simulink model "accBasedController_Simulation"  (R2020a)
settings: Solver=VariableStepAuto  StartTime=0  StopTime=20  FixedStep=0.001  RelTol=1e-3
values from neighbouring files (symbols this model uses):
  A = [0 0 5.53191489362 0 0 0 0 -107.82412766 0 221.276595745 0 1 ... (25 elements, 5x5)]    [CACu_ws.mat]    (also in SimulationParameters.m = [0 0 0 1 0 0;      0 0 0 0 1 0;      0 0 0 0 0 1;      -Ka/J; Simulation_ws.mat = [0 0 0 -118.993135011 5.87581816357 0 0 0 0 118.993135011 -1; abc_ws.mat = [0 0 0 1828.84460673 0 0 0 0 -1965.91569285 221.276595745 0 ; kalmanSS.m = [0 0 0 1 0 0;      0 0 0 0 1 0;      0 0 0 0 0 1;      -Ka/J)
  B = [1  0; 0  0; 0  0; 0  0; 0  19.2446808511]    [CACu_ws.mat]    (also in SimulationParameters.m = [zeros(3,control_dim); 1/Jh 0 0; 0 -1/Je 0; 0 0 N*KI/Ja]; Simulation_ws.mat = [0 0 0 22.8832951945 0 0 0 0 0 0 -1.12996503145 0 ... (18 el; abc_ws.mat = [1 0 0 0 0 0 0 0 -1.31799121269 0 0 0 ... (15 elements, 5x3); kalmanSS.m = [zeros(3,control_dim); 1/Jh 0 0; 0 -1/Je 0; 0 0 N*KI/Ja])
  C = [0 0 0 0 0 0 1 0 0 0 0 0 ... (25 elements, 5x5)]    [CACu_ws.mat]    (also in SimulationParameters.m = [zeros(sensor_dim,state_dim)]; Simulation_ws.mat = [-5.2 0 0 0 0 0 5.2 0 1 0 0 0 ... (36 elements, 6x6)]; abc_ws.mat; kalmanSS.m = [zeros(sensor_dim,state_dim)])
  CURRENT_MAX = 3.14    [CAC_ws.mat]    (also in CACu_ws.mat; SimulationParameters.m = 3.14159265359; Simulation_ws.mat = 3.14159265359; TransferFunctions.m = 3.14159265359)
  D = [1  0; 0  0; 0  0; 0  0; 0  0]    [CACu_ws.mat]    (also in SimulationParameters.m = zeros(sensor_dim, control_dim); Simulation_ws.mat = [0 0 0 0 0 0 0 0 0 0 0 0 ... (18 elements, 6x3)]; abc_ws.mat = [1 0 0 0 0 0 0 0 0 0 0 0 ... (15 elements, 5x3)]; kalmanSS.m = zeros(sensor_dim, control_dim))
  damping_d = 1.6    [CAC_ws.mat]    (also in CACu_ws.mat = 0.770835010154; abc_ws.mat = 0.770835010154; kalmanSSHumInput.m = 0.9; kalmanStateSpaceModellingHumInput.m = 0.9)
  dt = 0.001    [SimulationParameters.m]    (also in Simulation_ws.mat; TransferFunctions.m; kalmanSS.m; tests_analysis.m = 0.008)
  epos_Ki = 1.19    [CAC_ws.mat]    (also in CACu_ws.mat; TransferFunctions.m; abc_ws.mat; kalmanSSHumInput.m)
  epos_Kp = 11.9    [CAC_ws.mat]    (also in CACu_ws.mat; TransferFunctions.m; abc_ws.mat; kalmanSSHumInput.m)
  Fk = eye(state_dim) + A*dt + (A*dt)^2/prod(1:2) + (A*dt)^3/prod(1:3) + (A*dt)^4/prod(1:4)    [SimulationParameters.m]    (also in Simulation_ws.mat = [0.999940504052 2.93784973961e-06 5.41742100187e-11 -0.11899; kalmanSS.m)
  Gk = dt*(eye(state_dim) + A*dt/prod(1:2) + (A*dt)^2/prod(1:3) + (A*dt)^3/prod(1:4) +         (A*dt)^4/prod(1:5))*B    [SimulationParameters.m]    (also in Simulation_ws.mat = [1.14415341408e-05 5.60242006442e-12 0 0.0228828413715 2.240; kalmanSS.m = dt*(eye(state_dim) + A*dt/prod(1:2) + (A*dt)^2/prod(1:3) + ()
  I_zz = mass_scale*body_mass*(L_leg*r_zz)^2    (= 0.0437446334976)    [KneeJointParameters.m]    (also in SimulationParameters.m; Simulation_ws.mat; TransferFunctions.m; abc_ws.mat)
  Ja = 0.47    [CACu_ws.mat]    (also in SimulationParameters.m; Simulation_ws.mat; TransferFunctions.m; abc_ws.mat)
  Je = 0.94    [CACu_ws.mat]    (also in SimulationParameters.m = 0.88498313856; Simulation_ws.mat = 0.88498313856; TransferFunctions.m = 0.88498313856; abc_ws.mat = 0.7587304)
  Jh = 0.05    [CACu_ws.mat]    (also in SimulationParameters.m = 0.0437; Simulation_ws.mat = 0.0437; TransferFunctions.m = 0.0437; abc_ws.mat = 0.0437)
  Ka = 5.2    [CACu_ws.mat]    (also in SimulationParameters.m; Simulation_ws.mat; TransferFunctions.m = 6552; abc_ws.mat = 1387.6)
  KI = 0.0603    [CACu_ws.mat]    (also in SimulationParameters.m; Simulation_ws.mat; TransferFunctions.m; abc_ws.mat)
  Ks = 104    [CACu_ws.mat]    (also in SimulationParameters.m; Simulation_ws.mat; TransferFunctions.m; abc_ws.mat)
  Le = 0.4    [CACu_ws.mat]    (also in SimulationParameters.m = 0.432; Simulation_ws.mat = 0.432; TransferFunctions.m = 0.432; abc_ws.mat)
  N = 150    [CACu_ws.mat]    (also in SimulationParameters.m; Simulation_ws.mat; TransferFunctions.m; abc_ws.mat)
  Rk = eye(sensor_dim)    [kalmanStateSpaceModellingWithoutHum.m]
  sensor_dim = 5    [CACu_ws.mat]    (also in SimulationParameters.m = 6; Simulation_ws.mat = 6; abc_ws.mat; kalmanSS.m = 6)
  state_dim = 5    [CACu_ws.mat]    (also in SimulationParameters.m = 6; Simulation_ws.mat = 6; abc_ws.mat; kalmanSS.m = 6)
  stiffness_d = 1.04    [CAC_ws.mat]    (also in CACu_ws.mat = 14.0803237251; abc_ws.mat = 14.0803237251; kalmanSSHumInput.m = 3.874; kalmanStateSpaceModellingHumInput.m = 3.874)
  stiffness_lower = -20.9019922533    [CACu_ws.mat]    (also in abc_ws.mat; kalmanSSHumInput.m = -24.4873189611; kalmanStateSpaceModellingHumInput.m = -24.4873189611)
  Threaded_Ts = 0.001    [CAC_ws.mat]    (also in CACu_ws.mat; SimulationParameters.m; Simulation_ws.mat; abc_ws.mat)
  We = 19.6133    [CACu_ws.mat]    (also in SimulationParameters.m = 46.5037717323; Simulation_ws.mat = 46.5037717323; TransferFunctions.m = 46.5037717323; abc_ws.mat = 46.5037717323)
  zeta = 0.06    [SimulationParameters.m]    (also in Simulation_ws.mat; TransferFunctions.m; abc_ws.mat; kalmanSSHumInput.m = 0.01)
undefined symbols (not defined in the file or in its folder): A_kf, alpha, B_kf, C_kf, Continuous, D_kf, DiscIntNeverNeededParam, Discrete, gamma, k_bar, kf_ste_dim, nm_window, p_e_idx, p_m_idx, rho, sigma, Time, v_e_idx, v_h_idx, v_m_idx
libraries: simulink x23, dspstat3 x8, simulink_extras x5, ctrlSharedLib x2, dspsigops x2
(part 1 of 2)
Description:
  | Collocated Admittance Control study for the acceleration-based SEA Transparency Control
settings Model: OrderedModelArguments=off  Creator=Leonardo Felipe  LastModifiedBy=leona
settings DataIOCC: LimitDataPoints=on  MaxDataPoints=23000  SaveFormat=Array  InspectSignalLogs=on  ReturnWorkspaceOutputs=off
settings SFSimCC: CustomCodeUndefinedFunction=UseInterfaceOnly

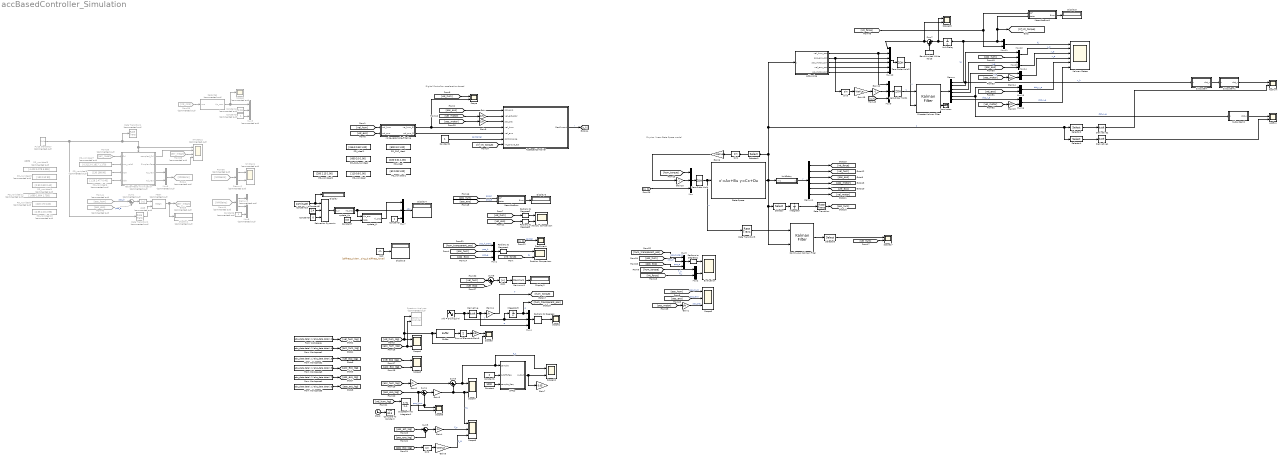
== system accBasedController_Simulation ==
  note: //RMS
  note: Digital Controller: acceleration-based
  note: Physics, linear State Space model
  Abs1 : Abs
  Abs3 : Abs  Commented=on
  AccBasedController : Subsystem  SystemSampleTime=dt
  AccExo : Scope  NumInputPorts=2
  AccHum : Scope  NumInputPorts=2
  Band-Limited White Noise : simulink/Sources/Band-Limited White Noise  Cov=2*5.476e-6  Ts=dt  seed=[23341]  VectorParams1D=off
  Buffer : Buffer  N=8  OutputFrames=off
  CAC : Constant  Value=[stiffness_d damping_d stiffness_lower]
  Clock : Clock
  Compare To Constant : simulink/Logic and Bit Operations/Compare To Constant  relop=<=  const=32.5  OutDataTypeStr=boolean
  Constant : Constant  Value=1000
  Constant1 : Constant  Value=2
  Constant10 : Constant  Value=sqrt(Ka/Je)
  Constant2 : Constant
  Constant3 : Constant  Commented=on
  Constant4 : Constant  Commented=on  Value=2.15
  Constant5 : Constant
  Constant6 : Constant  Commented=on
  Constant7 : Constant  Value=0.8
  Constant8 : Constant  Value=2.4
  Constant9 : Constant  Value=0
  Continuous Kalman Filter : ctrlSharedLib/Kalman Filter  TimeDomain=Continuous-Time  UseCurrentEstimator=on  ModelSource=LTI State-Space Variable  ModelSourceVariable=ss(A, B, C, D)  A=Fk  B=Gk  C=C  D=D  NumberOfStates=1  NumberOfInputs=1  NumberOfOutputs=1  InitialEstimateSource=Dialog  X0=zeros(state_dim,1)  P0=10  UseK=off  UseGH=off  NumberOfProcessNoiseInputs=1  G=1  TimeInvariantG=on  H=0  TimeInvariantH=on  Q=0.005*eye(state_dim)  TimeInvariantQ=on  R=0.01*eye(sensor_dim)  TimeInvariantR=on  N=0  TimeInvariantN=on  AddInputPort=on  AddEnablePort=off  OutputEstimatedY=off  OutputP=off  Ts=dt
  DIscrete Kalman Filter : ctrlSharedLib/Kalman Filter  TimeDomain=Discrete-Time  UseCurrentEstimator=on  ModelSource=Individual A, B, C, D matrices  ModelSourceVariable=ss(A_kf, B_kf, C_kf, D_kf)  A=Fk  B=Gk  C=C_kf  D=D_kf  NumberOfStates=1  NumberOfInputs=1  NumberOfOutputs=1  InitialEstimateSource=Dialog  X0=zeros(kf_ste_dim,1)  P0=10  UseK=off  UseGH=off  NumberOfProcessNoiseInputs=1  G=1  TimeInvariantG=on  H=0  TimeInvariantH=on  Q=Qk  TimeInvariantQ=on  R=Rk  TimeInvariantR=on  N=0  TimeInvariantN=on  AddInputPort=on  AddEnablePort=off  OutputEstimatedY=on  OutputP=off  Ts=dt
  Demux : Demux  Outputs=kf_ste_dim
  Demux1 : Demux  Outputs=6
  Demux2 : Demux  Commented=on  Outputs=2
  Demux3 : Demux  Commented=on  Outputs=2
  Derivative : Derivative
  Derivative1 : Derivative
  Derivative2 : Derivative
  DesCurrent : Scope
  Discrete-Time Integrator1 : DiscreteIntegrator  ExternalReset=level  InitialCondition=-0.16  SampleTime=dt  ICPrevOutput=DiscIntNeverNeededParam  ICPrevScaledInput=DiscIntNeverNeededParam
  Display{,2..6} (6 alike) : Display
  Display1 : Display  Commented=on
  Evaluation : Scope  NumInputPorts=2
  From Workspace : FromWorkspace  VariableName=[abc_data.data(:,1) abc_data.data(:,2)]  SampleTime=dt  OutputAfterFinalValue=Holding final value
  From Workspace1 : FromWorkspace  VariableName=[abc_data.data(:,1) abc_data.data(:,4)]  SampleTime=dt  OutputAfterFinalValue=Holding final value
  From Workspace2 : FromWorkspace  VariableName=[abc_data.data(:,1) abc_data.data(:,3)]  SampleTime=dt  OutputAfterFinalValue=Holding final value
  From Workspace3 : FromWorkspace  VariableName=[abc_data.data(:,1) abc_data.data(:,5)]  SampleTime=dt  OutputAfterFinalValue=Holding final value
  From Workspace4 : FromWorkspace  VariableName=[abc_data.data(:,1) abc_data.data(:,7)]  SampleTime=dt  OutputAfterFinalValue=Holding final value
  From Workspace5 : FromWorkspace  VariableName=[abc_data.data(:,1) abc_data.data(:,6)]  SampleTime=dt  OutputAfterFinalValue=Holding final value
  From35 : From  Commented=on  GotoTag=err_mean
  From36 : From  Commented=on  GotoTag=NMGains
  From38 : From  Commented=on  GotoTag=err_mean
  From39 : From  Commented=on  GotoTag=int_rms
  From40 : From  Commented=on  GotoTag=pos_exo
  From41 : From  Commented=on  GotoTag=pos_hum
  From44 : From  Commented=on  GotoTag=NMGains
  Gain{,1,8,13..14} (5 alike) : Gain  Gain=1/N
  Gain10 : Gain  Gain=-1
  Gain11 : Gain  Gain=Jh
  Gain12 : Gain  Gain=-1
  Gain15 : Gain  Gain=-We*Le
  Gain2 : Gain  Gain=Jh
  Gain3 : Gain  Gain=Ks/20
  Gain4 : Gain  Gain=Ks
  Gain5 : Gain  Gain=-We*Le
  Gain6 : Gain  Gain=-We*Le
  Gain7 : Gain  Gain=0.05
  Gain9 : Gain  Gain=1/8
  Goto4 : Goto  Commented=on  GotoTag=NMGains
  Goto5 : Goto  Commented=on  GotoTag=err_mean
  Integrator : Integrator
  Integrator3 : Integrator
  Kalman States : Scope  NumInputPorts=6
  LPF2p : Subsystem
  Maximum1 : dspstat3/Maximum  operation=maximum  fcn=Running  indexBase=One  operateOver=Each column  Dimension=1  InputProcessing=Columns as channels (frame based)  reset=None  roiEnable=off  roiType=Rectangles  roiPortion=Entire ROI  roiOutput=Individual statistics for each ROI  roiFlag=off  roundingMode=Floor  overflowMode=off  accumDataTypeStr=Inherit: Same as product output  accumLastDataTypeStr=Inherit: Same as product output
  Mean : dspstat3/Mean  Commented=on  run=on  InputProcessing=Columns as channels (frame based)  reset_popup=Falling edge  directionMode=Each column  dimension=1  roiEnable=off  roiType=Rectangles  roiPortion=Entire ROI  roiOutput=Individual statistics for each ROI  roiFlag=off  roundingMode=Floor  overflowMode=off  outputDataTypeStr=Inherit: Same as accumulator  outputMin=[]  outputMax=[]  outputLastDataTypeStr=Inherit: Same as accumulator
  MeanAbsError : Subsystem
  MeanAbsError1 : Subsystem
  Mux{,1,3..4,7,9} (6 alike) : Mux  Inputs=3
  Mux10 : Mux  Inputs=kf_snr_dim
  Mux{2,11..16} (7 alike) : Mux  Inputs=2
  Mux5 : Mux  Commented=on  Inputs=3
  Mux6 : Mux  Commented=on  Inputs=2
  Mux8 : Mux  Commented=on  Inputs=3
  NM Gains : Scope  Commented=on  NumInputPorts=2
  NM Status : Scope  Commented=on  NumInputPorts=4
  Nelder-Mead minimization : Subsystem  Commented=on  TreatAsAtomicUnit=on
  PD_CAC_ideal : Constant  Value=[600 3.0 1.00]
  PD_CAC_nonideal : Constant  Value=[600 3.0 1.00]
  PD_ideal : Constant  Value=[100 0.01 1.00]
  PD_ideal1 : Constant  Value=[246.9 0.60 1.00]
  PD_nonideal : Constant  Value=[110 0.8 1.00]
  PD_nonideal1 : Constant  Value=[60 0.08 1.00]
  PD_nonideal10 : Constant  Commented=on  Value=[2.55 2.15 2.95]  VectorParams1D=off
  PD_nonideal11 : Constant  Commented=on  Value=[1.699 1.604 1.758]
  PD_nonideal2 : Constant  Value=[200 2.15 1.00]
  PD_nonideal3 : Constant  Commented=on  Value=[130 110 90]
  PD_nonideal4 : Constant  Commented=on  Value=[0.90 0.80 0.40]  VectorParams1D=off
  PD_nonideal5 : Constant  Commented=on  Value=[130 188 90]
  PD_nonideal6 : Constant  Commented=on  Value=[1.29 2.477 0.40]  VectorParams1D=off
  PD_nonideal7 : Constant  Commented=on  Value=[0.3113 0.1817 1.170]
  PD_nonideal8 : Constant  Commented=on  Value=[4.423 5.078 6.355]
  PD_nonideal9 : Constant  Commented=on  Value=[220 170 240]
  Position Comparison : Scope  NumInputPorts=2
  Pulse Generator : DiscretePulseGenerator  Commented=on  PulseType=Time based  Period=nm_window  PulseWidth=5  PhaseDelay=0.95*nm_window
  Radians to Degrees{,1..4} (5 alike) : simulink_extras/Transformations/Radians to Degrees
  Rate Transition : RateTransition  OutPortSampleTime=dt
  Rate Transition1 : RateTransition  Commented=on
  Rate Transition2 : RateTransition  Commented=on
  Rate Transition3 : RateTransition
  Saturation Dynamic : simulink/Discontinuities/Saturation Dynamic  OutMin=[]  OutMax=[]  OutDataTypeStr=Inherit: Same as second input  OutDataType=fixdt(1, 16)  OutScaling=2^-10  DoSatur=off
  Scope{,3..5,7..8,10,17..18} (9 alike) : Scope  NumInputPorts=2
  Scope1 : Scope
  Scope2 : Scope  Commented=on
  Scope6 : Scope  NumInputPorts=3
  Scope9 : Scope  NumInputPorts=3
  Secantes : Subsystem  Commented=on  TreatAsAtomicUnit=on
  Selector : Selector  InputPortWidth=sensor_dim  IndexOptions=Index vector (dialog)  Indices=[v_h_idx]  OutputSizes=1
  Selector1 : Selector  InputPortWidth=sensor_dim  IndexOptions=Index vector (dialog)  Indices=[p_e_idx]  OutputSizes=1
  Selector2 : Selector  InputPortWidth=sensor_dim  IndexOptions=Index vector (dialog)  Indices=[v_h_idx]  OutputSizes=1
  Selector3 : Selector  InputPortWidth=state_dim  IndexOptions=Index vector (dialog)  Indices=[4]  OutputSizes=1
  Selector4 : Selector  InputPortWidth=sensor_dim  IndexOptions=Index vector (dialog)  Indices=[v_e_idx]  OutputSizes=1
  Sin1 : Trigonometry
  Sin2 : Trigonometry
  Sin3 : Trigonometry
  Spectrum Analyzer : SpectrumAnalyzer  Commented=on  NumInputPorts=2
  State-Space : StateSpace  A=A  B=B  C=C  D=D  InitialCondition=0  ContinuousStateAttributes={'x_h','x_e','x_a','dx_h','dx_e','dx_a'}
  Subsystem : Subsystem
  Subsystem1 : Subsystem
  Subsystem2 : Subsystem
  Sum of Elements : Sum  Inputs=+
  Sum1 : Sum  Commented=on  Inputs=|+-
  Sum{3..6} (4 alike) : Sum  Inputs=|+-
  Sum7 : Sum  Inputs=|++
  Terminator : Terminator
  Unit Delay : UnitDelay  SampleTime=-1  HasFrameUpgradeWarning=on
  UnitDelay : Subsystem  TreatAsAtomicUnit=on  SystemSampleTime=dt
  Velocity Comparison : Scope  NumInputPorts=2
  Zero-Order Hold : ZeroOrderHold  SampleTime=Threaded_Ts
  Zero-Order Hold1 : ZeroOrderHold  SampleTime=dt
  Zero-Order Hold2 : ZeroOrderHold  SampleTime=dt
  add_noise : Subsystem
  noise_resample_filtering : Subsystem
  update_Ki : Subsystem
  update_Kp : Subsystem
  w(t) = 3*sin(2pi*t) : Sin  Amplitude=3  Frequency=2*pi  SampleTime=0
  wires:
  Zero-Order Hold/1 -> Rate Transition3/1, State-Space/1  "u"
  State-Space/1 -> Selector4/1, Selector2/1, add_noise/1(y), Selector1/1, Selector/1, Continuous Kalman Filter/2, UnitDelay/1(In1)  "z"
  Mux/1 -> Zero-Order Hold/1
  UnitDelay/1(y) -> Demux1/1  "y"
  [vel_hum] -> Radians to Degrees2/1
  [vel_exo] -> Radians to Degrees3/1
  [pos_hum] -> Scope6/1  "pos_hum"
  [pos_exo] -> Scope6/2  "pos_exo"
  Constant2/1 -> AccBasedController/6(control_type)  "controller"
  [pos_exo] -> AccBasedController/1(pos_exo)
  [vel_motor] -> Gain/1
  Sin1/1 -> Gain6/1
  Demux1/3 -> [pos_exo]
  AccBasedController/1(DesCurrent) -> [u_k]  "I"
  Gain6/1 -> Gain10/1
  [pos_motor] -> Gain1/1
  Radians to Degrees2/1 -> Velocity Comparison/1
  Radians to Degrees3/1 -> Velocity Comparison/2
  [u_k] -> DesCurrent/1  "control"
  Gain10/1 -> Mux/2
  [vel_hum] -> Scope/1
  Demux1/2 -> [vel_hum]
  Demux1/1 -> [int_force]
  Demux1/4 -> [pos_motor]
  Demux1/5 -> [vel_exo]
  Demux1/6 -> [vel_motor]
  Mux1/1 -> Radians to Degrees4/1
  Radians to Degrees4/1 -> Position Comparison/1
  [int_force] -> Position Comparison/2  "t_i"
  [hum_torque] -> Mux/1
  Gain/1 -> AccBasedController/2(vel_actuator)
  Gain1/1 -> Scope6/3  "pos_act"
  From Workspace/1 -> [vel_hum_log]
  From Workspace1/1 -> [acc_hum_log]
  From Workspace3/1 -> [acc_exo_log]
  From Workspace2/1 -> [vel_exo_log]
  [acc_hum_log] -> Spectrum Analyzer/2, Scope4/2
  [vel_hum_log] -> Scope3/2, Buffer/1, Spectrum Analyzer/1, Scope4/1
  [acc_exo_log] -> Scope5/2
  [vel_exo_log] -> Scope5/1
  [acc_hum_log] -> Gain2/1
  Gain2/1 -> Sum3/1
  Sum4/1 -> Gain3/1
  Gain3/1 -> Sum3/2, Scope9/1, Scope7/2  "F_i"
  From Workspace4/1 -> [pos_exo_log]
  [pos_exo_log] -> Scope8/2, Sum4/1
  [vel_hum_log] -> Discrete-Time Integrator1/1
  Discrete-Time Integrator1/1 -> Sum4/2, Scope8/1  "pos_hum"
  Sum3/1 -> Scope10/1, LPF2p/1(sample), Scope7/1  "F_h"
  Clock/1 -> Compare To Constant/1
  From Workspace5/1 -> [pos_act_log]
  Sum5/1 -> Gain4/1
  [pos_act_log] -> Sum5/1
  [pos_exo_log] -> Sum5/2
  Gain4/1 -> Scope9/2  "F_s"
  Gain5/1 -> Scope9/3  "F_W"
  Sin2/1 -> Gain5/1
  [pos_exo_log] -> Sin2/1
  Constant/1 -> LPF2p/3(sample_freq)
  Constant1/1 -> LPF2p/2(cutoff_freq)
  LPF2p/1(output) -> Scope10/2, Gain7/1
  [vel_hum] -> Sum6/1
  [vel_exo] -> Sum6/2
  Abs1/1 -> Maximum1/1
  Maximum1/1 -> Display2/1
  Sum6/1 -> Abs1/1
  Gain8/1 -> AccBasedController/3(pos_act)
  [pos_motor] -> Gain8/1
  CAC/1 -> Display3/1
  Selector/1 -> Integrator/1
  Integrator/1 -> Rate Transition/1
  Rate Transition/1 -> [pos_hum]
  Selector1/1 -> Sin1/1
  [u_k] -> Mux/3
  [vel_hum] -> noise_resample_filtering/1(vel_hum)
  [vel_exo] -> noise_resample_filtering/2(vel_exo)
  noise_resample_filtering/1(ve_hum_filt) -> AccBasedController/4(vel_hum), Scope/2
  Mux3/1 -> Radians to Degrees1/1
  [pos_exo] -> Mux3/3  "pos_e"
  [pos_hum] -> Mux3/2  "pos_h"
  [hum_torque] -> Mux2/1  "T_h"
  [int_force] -> Mux2/2  "T_i"
  Mux2/1 -> Evaluation/2
  Radians to Degrees1/1 -> Evaluation/1
  [pos_exo] -> Mux1/3  "pos_e"
  [pos_hum] -> Mux1/2  "pos_h"
  [hum_transparent_pos] -> Mux1/1  "pos_h_trans"
  w(t) = 3*sin(2pi*t)/1 -> Integrator3/1, Mux4/2, Derivative/1  "v"
  Derivative/1 -> Mux4/3, Gain11/1  "a"
  Integrator3/1 -> [hum_transparent_pos], Mux4/1  "p"
  Mux4/1 -> Radians to Degrees/1
  Gain11/1 -> [hum_torque]  "T"
  Radians to Degrees/1 -> Scope1/1
  Constant3/1 -> Mux5/3
  From35/1 -> Nelder-Mead minimization/1(f(x))
  Pulse Generator/1 -> Rate Transition2/1, Rate Transition1/1, Nelder-Mead minimization/Trigger, NM Status/1
  PD_nonideal5/1 -> Nelder-Mead minimization/3(Kp0)
  PD_nonideal6/1 -> Nelder-Mead minimization/4(Kd0)
  PD_nonideal7/1 -> Nelder-Mead minimization/2(rms_vals0)
  Mux6/1 -> Goto4/1
  Nelder-Mead minimization/3(Kp_new) -> Mux6/1
  Nelder-Mead minimization/4(Kd_new) -> Mux6/2
  Nelder-Mead minimization/1(sampled_f(x)) -> NM Status/2
  From36/1 -> Demux2/1
  Demux2/1 -> NM Gains/1
  Demux2/2 -> NM Gains/2
  Nelder-Mead minimization/2(SimplexCase) -> NM Status/4
  From38/1 -> NM Status/3
  From39/1 -> Secantes/1(rms)
  Constant4/1 -> Mux5/2
  Secantes/1(Kp_new) -> Scope2/1, Mux5/1
  Constant5/1 -> Mux7/3
  From41/1 -> Sum1/1  "pos_h"
  From40/1 -> Sum1/2  "pos_e"
  Sum1/1 -> Abs3/1
  Abs3/1 -> Mean/1
  Mean/1 -> Display1/1, Goto5/1
  Rate Transition2/1 -> Mean/2
  Mux7/1 -> Display4/1  "Abc"
  Demux3/2 -> Mux8/2
  Demux3/1 -> Mux8/1
  Constant6/1 -> Mux8/3
  From44/1 -> Demux3/1
  update_Kp/1(Kp_acc) -> Mux7/2, update_Ki/1(Kp_acc)
  update_Ki/1(Ki_acc) -> Mux7/1
  Constant7/1 -> update_Ki/2(zeta)
  Constant9/1 -> Saturation Dynamic/3
  Constant8/1 -> Saturation Dynamic/2
  Saturation Dynamic/1 -> update_Kp/1(w_n)
  Constant10/1 -> Display/1, Saturation Dynamic/1
  [hum_transparent_pos] -> Mux3/1  "pos_h_trans"
  noise_resample_filtering/2(vel_exo_filt) -> AccBasedController/5(vel_exo)
  Buffer/1 -> Sum of Elements/1
  Sum of Elements/1 -> Gain9/1
  Gain9/1 -> Scope3/1
  add_noise/1(vel_hum_corr) -> Mux10/2, Mux9/1
  Gain12/1 -> Mux9/2
  Mux9/1 -> Zero-Order Hold1/1
  Zero-Order Hold1/1 -> DIscrete Kalman Filter/1  "u"
  [u_k] -> Mux9/3
  DIscrete Kalman Filter/1 -> Demux/1
  Mux10/1 -> Zero-Order Hold2/1
  add_noise/4(vel_exo_corr) -> Mux10/5
  Zero-Order Hold2/1 -> DIscrete Kalman Filter/2  "u"
  Rate Transition3/1 -> Continuous Kalman Filter/1
  Continuous Kalman Filter/1 -> Selector3/1
  Selector3/1 -> Scope17/1
  [vel_hum] -> Scope17/2
  [int_force] -> MeanAbsError1/1(ref), Mux11/2
  [pos_exo] -> Mux13/2
  Demux/3 -> Mux13/1  "x_e"
  Demux/1 -> MeanAbsError1/2(state), [kf_int_torque], Mux11/1, Unit Delay/1  "t_i"
  Demux/2 -> Mux12/1, Subsystem/1(x)  "x_h"
  [pos_hum] -> Mux12/2
  Demux/4 -> Mux14/1  "x_a"
  [pos_motor] -> Gain14/1
  Gain14/1 -> Mux14/2
  [vel_motor] -> Gain13/1
  [vel_exo] -> Mux15/2
  Demux/5 -> Mux15/1, Subsystem2/1(x)  "dot_x_e"
  Band-Limited White Noise/1 -> Sum7/2
  Sum7/1 -> Scope18/2, Mux10/1
  add_noise/2(pos_exo_corr) -> Sin3/1, Mux10/3
  add_noise/3(pos_motor_corr) -> Mux10/4
  add_noise/5(vel_motor_corr) -> Mux10/6
  Unit Delay/1 -> Scope18/1, Sum7/1
  Sin3/1 -> Gain15/1
  Gain15/1 -> Gain12/1
  Mux11/1 -> Kalman States/1  "t_i"
  Mux12/1 -> Kalman States/2  "x_h"
  Mux13/1 -> Kalman States/3  "x_e"
  Mux14/1 -> Kalman States/4  "x_a"
  Gain13/1 -> Mux16/2
  Demux/6 -> Mux16/1  "dot_x_a"
  Mux15/1 -> Kalman States/5  "dot_x_e"
  Mux16/1 -> Kalman States/6  "dot_x_a"
  [kf_int_torque] -> AccBasedController/7(int_torque_est)
  DIscrete Kalman Filter/2 -> Terminator/1
  Selector2/1 -> Derivative2/1
  Subsystem/1(dot_x) -> Subsystem1/1(x)
  Selector4/1 -> Derivative1/1
  [pos_hum] -> MeanAbsError/1(ref)  "pos_h"
  [pos_exo] -> MeanAbsError/2(state)  "pos_e"
  MeanAbsError/1(Error) -> Display6/1
  MeanAbsError1/1(Error) -> Display5/1
  Subsystem1/1(dot_x) -> AccHum/1
  Derivative2/1 -> AccHum/2
  Subsystem2/1(dot_x) -> AccExo/1
  Derivative1/1 -> AccExo/2

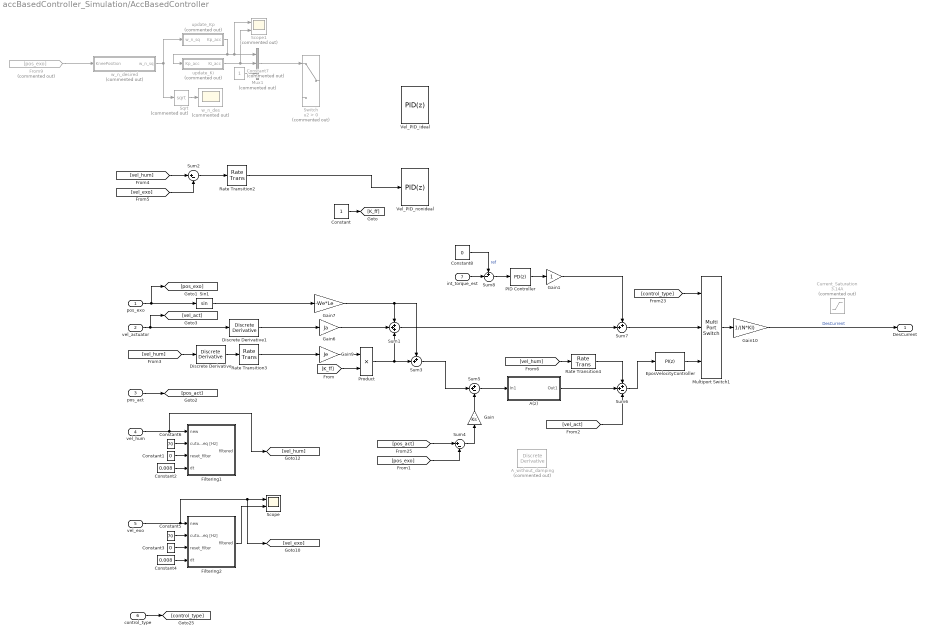
== system accBasedController_Simulation/AccBasedController ==
  pos_exo : Inport
  vel_actuator : Inport  Port=2
  pos_act : Inport  Port=3
  vel_hum : Inport  Port=4
  vel_exo : Inport  Port=5
  control_type : Inport  Port=6
  int_torque_est : Inport  Port=7
  A(z) : Subsystem
  A_without_damping : simulink/Discrete/Discrete Derivative  Commented=on  gainval=k_bar/stiffness_d  ICPrevScaledInput=0.0  OutMin=[]  OutMax=[]  OutDataType=fixdt(1, 16)  OutScaling=2^-10  DoSatur=off
  Constant : Constant
  Constant1 : Constant  Value=0
  Constant2 : Constant  Value=0.008
  Constant3 : Constant  Value=0
  Constant4 : Constant  Value=0.008
  Constant5 : Constant  Value=70
  Constant6 : Constant  Value=70
  Constant7 : Constant  Commented=on
  Constant8 : Constant  Value=0
  Current_Saturation 3.14A : Saturate  Commented=on  UpperLimit=CURRENT_MAX  LowerLimit=-CURRENT_MAX
  Discrete Derivative : simulink/Discrete/Discrete Derivative  gainval=1.0  ICPrevScaledInput=0.0  OutMin=[]  OutMax=[]  OutDataType=fixdt(1, 16)  OutScaling=2^-10  DoSatur=off
  Discrete Derivative1 : simulink/Discrete/Discrete Derivative  gainval=1.0  ICPrevScaledInput=0.0  OutMin=[]  OutMax=[]  OutDataType=fixdt(1, 16)  OutScaling=2^-10  DoSatur=off
  EposVelocityController : simulink/Continuous/PID Controller  Controller=PI  Form=Parallel  TimeDomain=Discrete-time  UseExternalTs=off  SampleTime=dt  IntegratorMethod=Forward Euler  FilterMethod=Forward Euler  ControllerParametersSource=internal  P=epos_Kp  I=epos_Ki  D=279.805559989798  UseFilter=off  N=100  TunerSelectOption=Transfer Function Based (PID Tuner App)  InitialConditionSource=internal  InitialConditionForIntegrator=0  InitialConditionForFilter=0  DifferentiatorICPrevScaledInput=0  ExternalReset=none  TrackingMode=off  Kt=1  LimitOutput=off  UpperSaturationLimit=inf  LowerSaturationLimit=-inf  LinearizeAsGain=on  AntiWindupMode=none  Kb=1  POutMin=[]  POutMax=[]  IOutMin=[]  IOutMax=[]  DOutMin=[]  DOutMax=[]  NOutMin=[]  NOutMax=[]  SumOutMin=[]  SumOutMax=[]  SaturationOutMin=[]  SaturationOutMax=[]  PParamMin=[]  PParamMax=[]  IParamMin=[]  IParamMax=[]  DParamMin=[]  DParamMax=[]  NParamMin=[]  NParamMax=[]  KbParamMin=[]  KbParamMax=[]  KtParamMin=[]  KtParamMax=[]  KbOutMin=[]  KbOutMax=[]  KtOutMin=[]  KtOutMax=[]  IntegratorOutMin=[]  IntegratorOutMax=[]  FilterOutMin=[]  FilterOutMax=[]  SumI1OutMin=[]  SumI1OutMax=[]  SumI2OutMin=[]  SumI2OutMax=[]  SumI3OutMin=[]  SumI3OutMax=[]  SumI4OutMin=[]  SumI4OutMax=[]  SumDOutMin=[]  SumDOutMax=[]  DifferentiatorOutMin=[]  DifferentiatorOutMax=[]  FilterDiffOutCoefMin=[]  FilterDiffOutCoefMax=[]  ReciprocalOutMin=[]  ReciprocalOutMax=[]  SumDenOutMin=[]  SumDenOutMax=[]  SumNumOutMin=[]  SumNumOutMax=[]  DivideOutMin=[]  DivideOutMax=[]  UdiffTsProdOutMin=[]  UdiffTsProdOutMax=[]  NTsProdOutMin=[]  NTsProdOutMax=[]  UintegralTsProdOutMin=[]  UintegralTsProdOutMax=[]  UngainTsProdOutMin=[]  UngainTsProdOutMax=[]  IntegratorContinuousStateAttributes=''  IntegratorStateMustResolveToSignalObject=off  IntegratorRTWStateStorageClass=Auto  FilterContinuousStateAttributes=''  FilterStateMustResolveToSignalObject=off  FilterRTWStateStorageClass=Auto  ParallelPVariant=InternalParameters  IdealPVariant=Disabled  IVariant=InternalParameters  DVariant=Disabled  IntegratorVariant=Discrete  SatVariant=Disabled  AWVariant=Passthrough  PCopyVariant=Disabled  TRVariant=Disabled  FdbkBlocksVariant=Forward  IdealPFdbkVariant=Disabled  SatFdbkVariant=Disabled  DerivativeFilterVariant=Disabled  NVariant=Disabled  NCopyVariant=Disabled_SignalSpec  FilterICVariant=Disabled  IntegratorICVariant=InternalICs  ExternalResetVariant=Disabled  TRSumVariant=Passthrough  SumFdbkVariant=Disabled  SumVariant=Sum_PI  TsampFilterVariant=InternalTs  TsampNgainVariant=Passthrough  TsampIntegralVariant=Passthrough
  Filtering1 : Subsystem
  Filtering2 : Subsystem
  From9 : From  Commented=on  GotoTag=pos_exo
  Gain : Gain  Gain=Ks
  Gain1 : Gain
  Gain10 : Gain  Gain=1/(N*KI)
  Gain6 : Gain  Gain=Ja
  Gain7 : Gain  Gain=-We*Le
  Gain9 : Gain  Gain=Je
  Multiport Switch1 : MultiPortSwitch  Inputs=2
  Mux1 : Mux  Commented=on  Inputs=3
  PID Controller : simulink/Continuous/PID Controller  Controller=PD  Form=Parallel  TimeDomain=Discrete-time  UseExternalTs=off  SampleTime=dt  IntegratorMethod=Forward Euler  FilterMethod=Forward Euler  ControllerParametersSource=internal  P=23  I=1  D=1.6  UseFilter=on  N=100  TunerSelectOption=Transfer Function Based (PID Tuner App)  InitialConditionSource=internal  InitialConditionForIntegrator=0  InitialConditionForFilter=0  DifferentiatorICPrevScaledInput=0  ExternalReset=none  TrackingMode=off  Kt=1  LimitOutput=off  UpperSaturationLimit=inf  LowerSaturationLimit=-inf  LinearizeAsGain=on  AntiWindupMode=none  Kb=1  POutMin=[]  POutMax=[]  IOutMin=[]  IOutMax=[]  DOutMin=[]  DOutMax=[]  NOutMin=[]  NOutMax=[]  SumOutMin=[]  SumOutMax=[]  SaturationOutMin=[]  SaturationOutMax=[]  PParamMin=[]  PParamMax=[]  IParamMin=[]  IParamMax=[]  DParamMin=[]  DParamMax=[]  NParamMin=[]  NParamMax=[]  KbParamMin=[]  KbParamMax=[]  KtParamMin=[]  KtParamMax=[]  KbOutMin=[]  KbOutMax=[]  KtOutMin=[]  KtOutMax=[]  IntegratorOutMin=[]  IntegratorOutMax=[]  FilterOutMin=[]  FilterOutMax=[]  SumI1OutMin=[]  SumI1OutMax=[]  SumI2OutMin=[]  SumI2OutMax=[]  SumI3OutMin=[]  SumI3OutMax=[]  SumI4OutMin=[]  SumI4OutMax=[]  SumDOutMin=[]  SumDOutMax=[]  DifferentiatorOutMin=[]  DifferentiatorOutMax=[]  FilterDiffOutCoefMin=[]  FilterDiffOutCoefMax=[]  ReciprocalOutMin=[]  ReciprocalOutMax=[]  SumDenOutMin=[]  SumDenOutMax=[]  SumNumOutMin=[]  SumNumOutMax=[]  DivideOutMin=[]  DivideOutMax=[]  UdiffTsProdOutMin=[]  UdiffTsProdOutMax=[]  NTsProdOutMin=[]  NTsProdOutMax=[]  UintegralTsProdOutMin=[]  UintegralTsProdOutMax=[]  UngainTsProdOutMin=[]  UngainTsProdOutMax=[]  IntegratorContinuousStateAttributes=''  IntegratorStateMustResolveToSignalObject=off  IntegratorRTWStateStorageClass=Auto  FilterContinuousStateAttributes=''  FilterStateMustResolveToSignalObject=off  FilterRTWStateStorageClass=Auto  ParallelPVariant=InternalParameters  IdealPVariant=Disabled  IVariant=Disabled  DVariant=InternalParameters  IntegratorVariant=Disabled  SatVariant=Disabled  AWVariant=Disabled  PCopyVariant=Disabled  TRVariant=Disabled  FdbkBlocksVariant=Forward  IdealPFdbkVariant=Disabled  SatFdbkVariant=Disabled  DerivativeFilterVariant=ForwardEulerFilter  NVariant=InternalParameters  NCopyVariant=Disabled  FilterICVariant=InternalICsFilter  IntegratorICVariant=Disabled  ExternalResetVariant=Disabled  TRSumVariant=Passthrough  SumFdbkVariant=Disabled  SumVariant=Sum_PD  TsampFilterVariant=InternalTs  TsampNgainVariant=Passthrough  TsampIntegralVariant=Disabled_SignalSpec
  Product : Product
  Rate Transition2 : RateTransition  OutPortSampleTime=0.001
  Rate Transition3 : RateTransition  OutPortSampleTime=0.001
  Rate Transition4 : RateTransition  OutPortSampleTime=0.001
  Scope : Scope  NumInputPorts=2
  Scope1 : Scope  Commented=on  NumInputPorts=2
  Sin1 : Trigonometry
  Sqrt : Sqrt  Commented=on  SaturateOnIntegerOverflow=on
  Sum1 : Sum  Inputs=+++
  Sum2 : Sum  Inputs=|+-
  Sum3 : Sum  Inputs=++|
  Sum4 : Sum  Inputs=|+-
  Sum5 : Sum  Inputs=++-
  Sum6 : Sum  Inputs=++-
  Sum7 : Sum  Inputs=++|
  Sum8 : Sum  Inputs=+-|
  Switch : Switch  Commented=on  Criteria=u2 > Threshold
  Vel_PID_ideal : simulink/Continuous/PID Controller  Controller=PID  Form=Parallel  TimeDomain=Discrete-time  UseExternalTs=off  SampleTime=dt  IntegratorMethod=Forward Euler  FilterMethod=Forward Euler  ControllerParametersSource=internal  P=340  I=289  D=0.034  UseFilter=off  N=100  TunerSelectOption=Transfer Function Based (PID Tuner App)  InitialConditionSource=internal  InitialConditionForIntegrator=0  InitialConditionForFilter=0  DifferentiatorICPrevScaledInput=0  ExternalReset=none  TrackingMode=off  Kt=1  LimitOutput=off  UpperSaturationLimit=inf  LowerSaturationLimit=-inf  LinearizeAsGain=on  AntiWindupMode=none  Kb=1  POutMin=[]  POutMax=[]  IOutMin=[]  IOutMax=[]  DOutMin=[]  DOutMax=[]  NOutMin=[]  NOutMax=[]  SumOutMin=[]  SumOutMax=[]  SaturationOutMin=[]  SaturationOutMax=[]  PParamMin=[]  PParamMax=[]  IParamMin=[]  IParamMax=[]  DParamMin=[]  DParamMax=[]  NParamMin=[]  NParamMax=[]  KbParamMin=[]  KbParamMax=[]  KtParamMin=[]  KtParamMax=[]  KbOutMin=[]  KbOutMax=[]  KtOutMin=[]  KtOutMax=[]  IntegratorOutMin=[]  IntegratorOutMax=[]  FilterOutMin=[]  FilterOutMax=[]  SumI1OutMin=[]  SumI1OutMax=[]  SumI2OutMin=[]  SumI2OutMax=[]  SumI3OutMin=[]  SumI3OutMax=[]  SumI4OutMin=[]  SumI4OutMax=[]  SumDOutMin=[]  SumDOutMax=[]  DifferentiatorOutMin=[]  DifferentiatorOutMax=[]  FilterDiffOutCoefMin=[]  FilterDiffOutCoefMax=[]  ReciprocalOutMin=[]  ReciprocalOutMax=[]  SumDenOutMin=[]  SumDenOutMax=[]  SumNumOutMin=[]  SumNumOutMax=[]  DivideOutMin=[]  DivideOutMax=[]  UdiffTsProdOutMin=[]  UdiffTsProdOutMax=[]  NTsProdOutMin=[]  NTsProdOutMax=[]  UintegralTsProdOutMin=[]  UintegralTsProdOutMax=[]  UngainTsProdOutMin=[]  UngainTsProdOutMax=[]  IntegratorContinuousStateAttributes=''  IntegratorStateMustResolveToSignalObject=off  IntegratorRTWStateStorageClass=Auto  FilterContinuousStateAttributes=''  FilterStateMustResolveToSignalObject=off  FilterRTWStateStorageClass=Auto  ParallelPVariant=InternalParameters  IdealPVariant=Disabled  IVariant=InternalParameters  DVariant=InternalParameters  IntegratorVariant=Discrete  SatVariant=Disabled  AWVariant=Passthrough  PCopyVariant=Disabled  TRVariant=Disabled  FdbkBlocksVariant=Forward  IdealPFdbkVariant=Disabled  SatFdbkVariant=Disabled  DerivativeFilterVariant=Differentiator  NVariant=Passthrough  NCopyVariant=Disabled_SignalSpec  FilterICVariant=InternalICsDifferentiator  IntegratorICVariant=InternalICs  ExternalResetVariant=Disabled  TRSumVariant=Passthrough  SumFdbkVariant=Disabled  SumVariant=Sum_PID  TsampFilterVariant=InternalTs  TsampNgainVariant=Passthrough  TsampIntegralVariant=Passthrough
  Vel_PID_nonideal : simulink/Continuous/PID Controller  Controller=PID  Form=Parallel  TimeDomain=Discrete-time  UseExternalTs=off  SampleTime=dt  IntegratorMethod=Forward Euler  FilterMethod=Forward Euler  ControllerParametersSource=internal  P=1.7  I=195.5  D=0.459  UseFilter=off  N=100  TunerSelectOption=Transfer Function Based (PID Tuner App)  InitialConditionSource=internal  InitialConditionForIntegrator=0  InitialConditionForFilter=0  DifferentiatorICPrevScaledInput=0  ExternalReset=none  TrackingMode=off  Kt=1  LimitOutput=off  UpperSaturationLimit=inf  LowerSaturationLimit=-inf  LinearizeAsGain=on  AntiWindupMode=none  Kb=1  POutMin=[]  POutMax=[]  IOutMin=[]  IOutMax=[]  DOutMin=[]  DOutMax=[]  NOutMin=[]  NOutMax=[]  SumOutMin=[]  SumOutMax=[]  SaturationOutMin=[]  SaturationOutMax=[]  PParamMin=[]  PParamMax=[]  IParamMin=[]  IParamMax=[]  DParamMin=[]  DParamMax=[]  NParamMin=[]  NParamMax=[]  KbParamMin=[]  KbParamMax=[]  KtParamMin=[]  KtParamMax=[]  KbOutMin=[]  KbOutMax=[]  KtOutMin=[]  KtOutMax=[]  IntegratorOutMin=[]  IntegratorOutMax=[]  FilterOutMin=[]  FilterOutMax=[]  SumI1OutMin=[]  SumI1OutMax=[]  SumI2OutMin=[]  SumI2OutMax=[]  SumI3OutMin=[]  SumI3OutMax=[]  SumI4OutMin=[]  SumI4OutMax=[]  SumDOutMin=[]  SumDOutMax=[]  DifferentiatorOutMin=[]  DifferentiatorOutMax=[]  FilterDiffOutCoefMin=[]  FilterDiffOutCoefMax=[]  ReciprocalOutMin=[]  ReciprocalOutMax=[]  SumDenOutMin=[]  SumDenOutMax=[]  SumNumOutMin=[]  SumNumOutMax=[]  DivideOutMin=[]  DivideOutMax=[]  UdiffTsProdOutMin=[]  UdiffTsProdOutMax=[]  NTsProdOutMin=[]  NTsProdOutMax=[]  UintegralTsProdOutMin=[]  UintegralTsProdOutMax=[]  UngainTsProdOutMin=[]  UngainTsProdOutMax=[]  IntegratorContinuousStateAttributes=''  IntegratorStateMustResolveToSignalObject=off  IntegratorRTWStateStorageClass=Auto  FilterContinuousStateAttributes=''  FilterStateMustResolveToSignalObject=off  FilterRTWStateStorageClass=Auto  ParallelPVariant=InternalParameters  IdealPVariant=Disabled  IVariant=InternalParameters  DVariant=InternalParameters  IntegratorVariant=Discrete  SatVariant=Disabled  AWVariant=Passthrough  PCopyVariant=Disabled  TRVariant=Disabled  FdbkBlocksVariant=Forward  IdealPFdbkVariant=Disabled  SatFdbkVariant=Disabled  DerivativeFilterVariant=Differentiator  NVariant=Passthrough  NCopyVariant=Disabled_SignalSpec  FilterICVariant=InternalICsDifferentiator  IntegratorICVariant=InternalICs  ExternalResetVariant=Disabled  TRSumVariant=Passthrough  SumFdbkVariant=Disabled  SumVariant=Sum_PID  TsampFilterVariant=InternalTs  TsampNgainVariant=Passthrough  TsampIntegralVariant=Passthrough
  update_Ki : Subsystem  Commented=on
  update_Kp : Subsystem  Commented=on
  w_n_des : Scope  Commented=on
  w_n_desired : Subsystem  Commented=on
  DesCurrent : Outport
  wires:
  Gain7/1 -> Sum3/1, Sum1/1
  Multiport Switch1/1 -> Gain10/1
  Rate Transition3/1 -> Gain9/1
  pos_exo/1 -> [pos_exo], Sin1/1
  vel_actuator/1 -> [vel_act], Discrete Derivative1/1
  [control_type] -> Multiport Switch1/1
  Sin1/1 -> Gain7/1
  control_type/1 -> [control_type]
  Product/1 -> Sum3/2, Sum1/3
  Discrete Derivative1/1 -> Gain6/1
  Rate Transition2/1 -> Vel_PID_nonideal/1
  [K_ff] -> Product/2
  Gain9/1 -> Product/1
  Constant4/1 -> Filtering2/4(dt)
  Constant5/1 -> Filtering2/2(cutoff_freq [Hz])
  Constant3/1 -> Filtering2/3(reset_filter)
  vel_exo/1 -> [vel_exo], Scope/1, Filtering2/1(new)
  vel_hum/1 -> [vel_hum], Filtering1/1(new)
  Constant1/1 -> Filtering1/3(reset_filter)
  Constant6/1 -> Filtering1/2(cutoff_freq [Hz])
  Constant2/1 -> Filtering1/4(dt)
  Sqrt/1 -> w_n_des/1
  From9/1 -> w_n_desired/1(KneePosition)
  Constant7/1 -> Mux1/3
  update_Kp/1(Kp_acc) -> update_Ki/1(Kp_acc), Scope1/1, Mux1/1
  w_n_desired/1(w_n_sq) -> update_Kp/1(w_n_sq), Sqrt/1
  update_Ki/1(Ki_acc) -> Mux1/2, Scope1/2
  Mux1/1 -> Switch/1
  Sum2/1 -> Rate Transition2/1
  Discrete Derivative/1 -> Rate Transition3/1
  Gain6/1 -> Sum1/2
  Gain10/1 -> DesCurrent/1  "DesCurrent"
  EposVelocityController/1 -> Multiport Switch1/3
  Sum7/1 -> Multiport Switch1/2
  pos_act/1 -> [pos_act]
  [pos_act] -> Sum4/1
  [pos_exo] -> Sum4/2
  Sum4/1 -> Gain/1
  Sum1/1 -> Sum7/2
  Sum6/1 -> EposVelocityController/1
  Filtering2/1(filtered) -> Scope/2
  [vel_hum] -> Discrete Derivative/1
  [vel_hum] -> Sum2/1
  [vel_exo] -> Sum2/2
  [vel_act] -> Sum6/3
  [vel_hum] -> Rate Transition4/1
  Rate Transition4/1 -> Sum6/1
  A(z)/1(Out1) -> Sum6/2
  Gain/1 -> Sum5/3
  Sum3/1 -> Sum5/2
  Sum5/1 -> A(z)/1(In1)
  Constant/1 -> [K_ff]
  int_torque_est/1 -> Sum8/2
  Sum8/1 -> PID Controller/1
  Constant8/1 -> Sum8/1  "ref"
  PID Controller/1 -> Gain1/1
  Gain1/1 -> Sum7/1

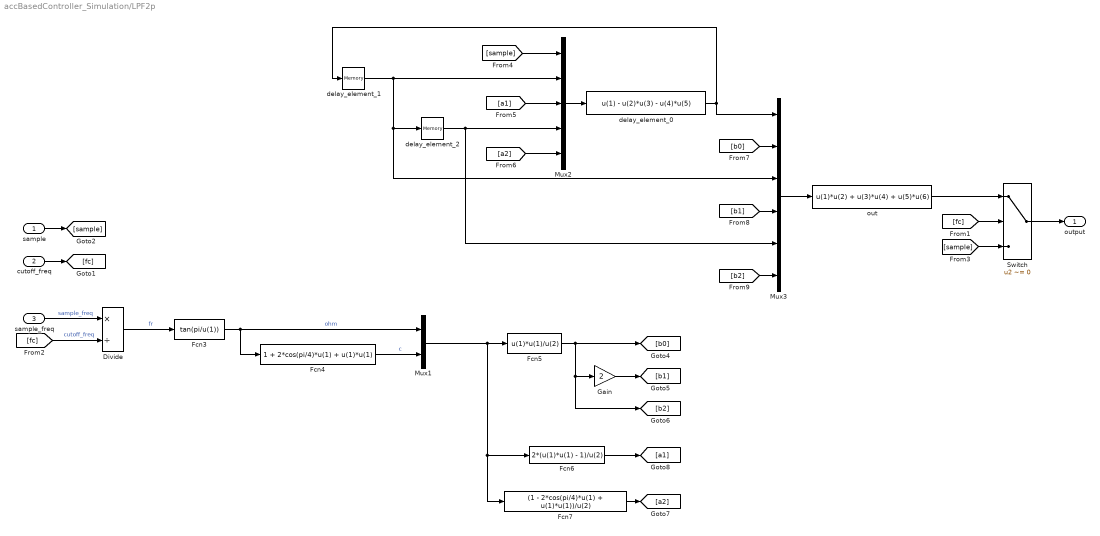
== system accBasedController_Simulation/LPF2p ==
  sample : Inport
  cutoff_freq : Inport  Port=2
  sample_freq : Inport  Port=3
  Divide : Product  Inputs=*/
  Fcn3 : Fcn  Expr=tan(pi/u(1))
  Fcn4 : Fcn  Expr=1 + 2*cos(pi/4)*u(1) + u(1)*u(1)
  Fcn5 : Fcn  Expr=u(1)*u(1)/u(2)
  Fcn6 : Fcn  Expr=2*(u(1)*u(1) - 1)/u(2)
  Fcn7 : Fcn  Expr=(1 - 2*cos(pi/4)*u(1) + u(1)*u(1))/u(2)
  Gain : Gain  Gain=2
  Mux1 : Mux  Inputs=2
  Mux2 : Mux  Inputs=5
  Mux3 : Mux  Inputs=6
  Switch : Switch  Criteria=u2 ~= 0
  delay_element_0 : Fcn  Expr=u(1) - u(2)*u(3) - u(4)*u(5)
  delay_element_1 : Memory  InheritSampleTime=on
  delay_element_2 : Memory  InheritSampleTime=on
  out : Fcn  Expr=u(1)*u(2) + u(3)*u(4) + u(5)*u(6)
  output : Outport
  wires:
  Switch/1 -> output/1
  cutoff_freq/1 -> [fc]
  [fc] -> Switch/2
  sample_freq/1 -> Divide/1  "sample_freq"
  [fc] -> Divide/2  "cutoff_freq"
  Divide/1 -> Fcn3/1  "fr"
  Mux1/1 -> Fcn7/1, Fcn6/1, Fcn5/1
  Fcn3/1 -> Mux1/1, Fcn4/1  "ohm"
  Fcn4/1 -> Mux1/2  "c"
  Fcn5/1 -> [b0], [b2], Gain/1
  Gain/1 -> [b1]
  Fcn6/1 -> [a1]
  Fcn7/1 -> [a2]
  sample/1 -> [sample]
  [sample] -> Switch/3
  delay_element_1/1 -> delay_element_2/1, Mux3/3, Mux2/2
  [sample] -> Mux2/1
  Mux2/1 -> delay_element_0/1
  [a1] -> Mux2/3
  delay_element_2/1 -> Mux2/4, Mux3/5
  [a2] -> Mux2/5
  out/1 -> Switch/1
  delay_element_0/1 -> delay_element_1/1, Mux3/1
  [b0] -> Mux3/2
  [b1] -> Mux3/4
  [b2] -> Mux3/6
  Mux3/1 -> out/1

== system accBasedController_Simulation/MeanAbsError ==
  ref : Inport
  state : Inport  Port=2
  Abs4 : Abs
  Mean1 : dspstat3/Mean  run=on  InputProcessing=Columns as channels (frame based)  reset_popup=None  directionMode=Each column  dimension=1  roiEnable=off  roiType=Rectangles  roiPortion=Entire ROI  roiOutput=Individual statistics for each ROI  roiFlag=off  roundingMode=Floor  overflowMode=off  outputDataTypeStr=Inherit: Same as accumulator  outputMin=[]  outputMax=[]  outputLastDataTypeStr=Inherit: Same as accumulator
  Sum2 : Sum  Inputs=|+-
  Error : Outport
  wires:
  state/1 -> Sum2/2
  Abs4/1 -> Mean1/1
  Sum2/1 -> Abs4/1
  Mean1/1 -> Error/1
  ref/1 -> Sum2/1

== system accBasedController_Simulation/MeanAbsError1 ==
  ref : Inport
  state : Inport  Port=2
  Abs4 : Abs
  Mean1 : dspstat3/Mean  run=on  InputProcessing=Columns as channels (frame based)  reset_popup=None  directionMode=Each column  dimension=1  roiEnable=off  roiType=Rectangles  roiPortion=Entire ROI  roiOutput=Individual statistics for each ROI  roiFlag=off  roundingMode=Floor  overflowMode=off  outputDataTypeStr=Inherit: Same as accumulator  outputMin=[]  outputMax=[]  outputLastDataTypeStr=Inherit: Same as accumulator
  Sum2 : Sum  Inputs=|+-
  Error : Outport
  wires:
  ref/1 -> Sum2/1
  Mean1/1 -> Error/1
  Sum2/1 -> Abs4/1
  Abs4/1 -> Mean1/1
  state/1 -> Sum2/2

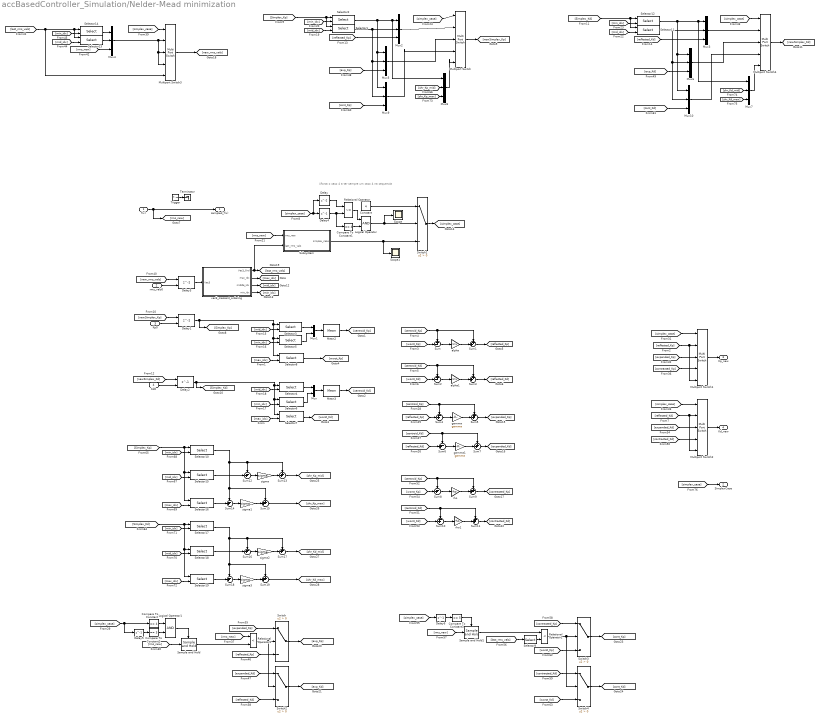
== system accBasedController_Simulation/Nelder-Mead minimization ==
  note: //forca o caso 4 a ter sempre um caso 4 na sequencia
  f(x) : Inport
  rms_vals0 : Inport  Port=2
  Kp0 : Inport  Port=3
  Kd0 : Inport  Port=4
  Trigger : TriggerPort  VariantControl=Variant  ShowOutputPort=on  OutputDataType=int8
  Compare To Constant : simulink/Logic and Bit Operations/Compare To Constant  relop===  const=4  OutDataTypeStr=boolean
  Compare To Constant1 : simulink/Logic and Bit Operations/Compare To Constant  relop===  const=4  OutDataTypeStr=boolean
  Compare To Constant2 : simulink/Logic and Bit Operations/Compare To Constant  relop===  const=3  OutDataTypeStr=boolean
  Compare To Constant3 : simulink/Logic and Bit Operations/Compare To Constant  relop===  const=5  OutDataTypeStr=boolean
  Constant : Constant  Value=4
  Delay : Delay
  Delay1 : Delay  DelayLength=1  InitialConditionSource=Input port
      settings: InputPortMap=u0,p4
  Delay2 : Delay  DelayLength=1  InitialConditionSource=Input port
      settings: InputPortMap=u0,p4
  Delay3 : Delay  DelayLength=1  InitialConditionSource=Input port
      settings: InputPortMap=u0,p4
  Delay4 : Delay  DelayLength=1
  Delay5 : Delay  DelayLength=1
  Delay6 : Delay  DelayLength=1
  Logical Operator : Logic  AllPortsSameDT=off  OutDataTypeStr=boolean
  Logical Operator1 : Logic  AllPortsSameDT=off  OutDataTypeStr=boolean
  Mean2 : dspstat3/Mean  run=off  InputProcessing=Columns as channels (frame based)  reset_popup=None  directionMode=Each column  dimension=1  roiEnable=off  roiType=Rectangles  roiPortion=Entire ROI  roiOutput=Individual statistics for each ROI  roiFlag=off  roundingMode=Floor  overflowMode=off  outputDataTypeStr=Inherit: Same as accumulator  outputMin=[]  outputMax=[]  outputLastDataTypeStr=Inherit: Same as accumulator
  Mean3 : dspstat3/Mean  run=off  InputProcessing=Columns as channels (frame based)  reset_popup=None  directionMode=Each column  dimension=1  roiEnable=off  roiType=Rectangles  roiPortion=Entire ROI  roiOutput=Individual statistics for each ROI  roiFlag=off  roundingMode=Floor  overflowMode=off  outputDataTypeStr=Inherit: Same as accumulator  outputMin=[]  outputMax=[]  outputLastDataTypeStr=Inherit: Same as accumulator
  Multiport Switch{,1..4} (5 alike) : MultiPortSwitch  DataPortOrder=Specify indices  DataPortIndices={3,4,5,6}  DiagnosticForDefault=Warning
  Mux : Mux  Inputs=2
  Mux1 : Mux  Inputs=2
  Mux{2..10} (9 alike) : Mux  Inputs=3
  Relational Operator : RelationalOperator  Operator=~=  OutDataTypeStr=boolean  RndMeth=Simplest
  Relational Operator1 : RelationalOperator  Operator=<  OutDataTypeStr=boolean  RndMeth=Simplest
  Relational Operator3 : RelationalOperator  Operator=<  OutDataTypeStr=boolean  RndMeth=Simplest
  Sample and Hold : dspsigops/Sample and Hold  trig=Rising edge  initCond=0  latchinput=off
  Sample and Hold1 : dspsigops/Sample and Hold  trig=Rising edge  initCond=0  latchinput=off
  Scope : Scope
  Scope1 : Scope
  Selector{1..8,10..19} (18 alike) : Selector  InputPortWidth=3  IndexOptions=Index vector (port)  Indices=[1]  OutputSizes=1
  Selector9 : Selector  InputPortWidth=3  IndexOptions=Index vector (dialog)  Indices=[3]  OutputSizes=1
  Subsystem : Subsystem
  Sum : Sum  Inputs=+-|
  Sum{1,3,5,7,9,11,13,15,17,19} (10 alike) : Sum  Inputs=++|
  Sum{4,6,8,10,12,14,16,18} (8 alike) : Sum  Inputs=-+|
  Sum2 : Sum  Inputs=+-|
  Switch{,1..4} (5 alike) : Switch  Criteria=u2 > Threshold
  Terminator : Terminator
  alpha : Gain  Gain=alpha
  alpha1 : Gain  Gain=alpha
  gamma : Gain  Gain=gamma
  gamma1 : Gain  Gain=gamma
  rho : Gain  Gain=rho
  rho1 : Gain  Gain=rho
  sigma{,1..3} (4 alike) : Gain  Gain=sigma
  vec3_crescent_ordering : Subsystem
  sampled_f(x) : Outport  SourceOfInitialOutputValue=Input signal
  SimplexCase : Outport  Port=2
  Kp_new : Outport  Port=3  SourceOfInitialOutputValue=Input signal
  Kd_new : Outport  Port=4  SourceOfInitialOutputValue=Input signal
  wires:
  f(x)/1 -> [rms_new], sampled_f(x)/1
  Trigger/1 -> Terminator/1
  Delay1/1 -> [Simplex_Kp], Selector8/1, Selector5/1, Selector3/1
  Delay2/1 -> [Simplex_Kd], Selector7/1, Selector6/1, Selector4/1
  vec3_crescent_ordering/4(min_idx) -> [min_idx]
  Selector4/1 -> Mux/1
  Selector6/1 -> Mux/2
  Selector3/1 -> Mux1/1
  Selector5/1 -> Mux1/2
  Mux1/1 -> Mean2/1
  Mux/1 -> Mean3/1
  vec3_crescent_ordering/2(max_idx) -> [max_idx]
  [max_idx] -> Selector7/2
  [max_idx] -> Selector8/2
  Mean2/1 -> [centroid_Kp]
  Mean3/1 -> [centroid_Kd]
  Selector7/1 -> [worst_Kd]
  Selector8/1 -> [worst_Kp]
  [centroid_Kp] -> Sum1/1, Sum/1
  [worst_Kp] -> Sum/2
  Sum/1 -> alpha/1
  alpha/1 -> Sum1/2
  alpha1/1 -> Sum3/2
  Sum2/1 -> alpha1/1
  [worst_Kd] -> Sum2/2
  [centroid_Kd] -> Sum2/1, Sum3/1
  Sum1/1 -> [reflected_Kp]
  Sum3/1 -> [reflected_Kd]
  Kp0/1 -> Delay1/2
  Kd0/1 -> Delay2/2
  rms_vals0/1 -> Delay3/2
  Delay3/1 -> vec3_crescent_ordering/1(Vec3)
  [newSimplex_Kp] -> Delay1/1
  [newSimplex_Kd] -> Delay2/1
  [min_idx] -> Selector5/2
  [min_idx] -> Selector6/2
  vec3_crescent_ordering/3(middle_idx) -> [mid_idx]
  [mid_idx] -> Selector3/2
  [mid_idx] -> Selector4/2
  [mid_idx] -> Selector1/2
  [min_idx] -> Selector2/2
  Selector2/1 -> Mux8/1, Mux2/1, Mux5/1, Mux9/1
  Selector1/1 -> Mux2/2, Mux5/2, Mux9/2
  [Simplex_Kp] -> Selector1/1, Selector2/1
  [Simplex_Kd] -> Selector12/1, Selector11/1
  Selector11/1 -> Mux3/2, Mux6/2, Mux10/2
  Selector12/1 -> Mux7/1, Mux3/1, Mux10/1, Mux6/1
  [min_idx] -> Selector12/2
  [mid_idx] -> Selector11/2
  [simplex_case] -> Multiport Switch/1
  [centroid_Kp] -> Sum5/1, Sum4/1
  Sum4/1 -> gamma/1
  gamma/1 -> Sum5/2
  [reflected_Kp] -> Sum4/2
  Sum5/1 -> [expanded_Kp]
  Sum7/1 -> [expanded_Kd]
  [reflected_Kd] -> Sum6/2
  gamma1/1 -> Sum7/2
  Sum6/1 -> gamma1/1
  [centroid_Kd] -> Sum6/1, Sum7/1
  [simplex_case] -> Compare To Constant/1, Delay5/1
  [rms_new] -> Sample and Hold/1
  [simplex_case] -> Multiport Switch1/1
  [reflected_Kp] -> Multiport Switch1/5, Multiport Switch1/2
  [expanded_Kp] -> Multiport Switch1/3
  Multiport Switch1/1 -> Kp_new/1
  [simplex_case] -> Multiport Switch2/1
  Multiport Switch2/1 -> Kd_new/1
  [reflected_Kd] -> Multiport Switch2/5, Multiport Switch2/2
  [expanded_Kd] -> Multiport Switch2/3
  Delay4/1 -> Relational Operator/2, Compare To Constant1/1
  [new_rms_vals] -> Delay3/1
  [simplex_case] -> Multiport Switch3/1
  Multiport Switch3/1 -> [new_rms_vals]
  vec3_crescent_ordering/1(Vec3_Ord) -> Subsystem/2(last_rms_vals), [last_rms_vals]
  [simplex_case] -> Multiport Switch4/1
  [rms_new] -> Relational Operator3/1
  Sample and Hold/1 -> Relational Operator3/2
  Relational Operator3/1 -> Switch2/2, Switch/2
  [rms_new] -> Subsystem/1(rms_new)
  Mux4/1 -> Multiport Switch3/4, Multiport Switch3/3, Multiport Switch3/2
  [last_rms_vals] -> Multiport Switch3/5, Selector14/1, Selector13/1
  Selector13/1 -> Mux4/2
  Selector14/1 -> Mux4/1
  [min_idx] -> Selector14/2
  [mid_idx] -> Selector13/2
  [rms_new] -> Mux4/3
  Multiport Switch4/1 -> [newSimplex_Kd]
  [reflected_Kd] -> Mux3/3
  Mux3/1 -> Multiport Switch4/2
  [reflected_Kp] -> Mux2/3
  Multiport Switch/1 -> [newSimplex_Kp]
  Mux2/1 -> Multiport Switch/2
  Switch1/1 -> [simplex_case]
  Subsystem/1(simplex_case) -> Scope1/1, Switch1/3
  Constant/1 -> Switch1/1
  Logical Operator/1 -> Scope/1, Switch1/2
  Compare To Constant1/1 -> Logical Operator/2
  [simplex_case] -> Delay/1, Delay4/1
  Relational Operator/1 -> Logical Operator/1
  Delay/1 -> Relational Operator/1
  Compare To Constant/1 -> Logical Operator1/1
  Delay5/1 -> Compare To Constant2/1
  Compare To Constant2/1 -> Logical Operator1/2
  Logical Operator1/1 -> Sample and Hold/Trigger
  Switch/1 -> [exp_Kp]
  [expanded_Kp] -> Switch/1
  [reflected_Kd] -> Switch2/3
  Switch2/1 -> [exp_Kd]
  [reflected_Kp] -> Switch/3
  [expanded_Kd] -> Switch2/1
  Mux5/1 -> Multiport Switch/3
  [exp_Kp] -> Mux5/3
  Mux6/1 -> Multiport Switch4/3
  [exp_Kd] -> Mux6/3
  Mux7/1 -> Multiport Switch4/5
  Mux8/1 -> Multiport Switch/5
  [centroid_Kd] -> Sum11/1, Sum10/1
  Sum10/1 -> rho1/1
  rho1/1 -> Sum11/2
  [worst_Kd] -> Sum10/2
  Sum11/1 -> [contracted_Kd]
  Sum9/1 -> [contracted_Kp]
  [worst_Kp] -> Sum8/2
  rho/1 -> Sum9/2
  Sum8/1 -> rho/1
  [centroid_Kp] -> Sum8/1, Sum9/1
  [contracted_Kp] -> Multiport Switch1/4
  [contracted_Kd] -> Multiport Switch2/4
  [simplex_case] -> Delay6/1
  Delay6/1 -> Compare To Constant3/1
  [last_rms_vals] -> Selector9/1
  Compare To Constant3/1 -> Sample and Hold1/Trigger
  [rms_new] -> Sample and Hold1/1
  Sample and Hold1/1 -> Relational Operator1/1
  Selector9/1 -> Relational Operator1/2
  Relational Operator1/1 -> Switch4/2, Switch3/2
  Switch3/1 -> [cont_Kp]
  [contracted_Kp] -> Switch3/1
  Switch4/1 -> [cont_Kd]
  [contracted_Kd] -> Switch4/1
  [worst_Kp] -> Switch3/3
  [worst_Kd] -> Switch4/3
  Mux9/1 -> Multiport Switch/4
  [cont_Kp] -> Mux9/3
  Mux10/1 -> Multiport Switch4/4
  [cont_Kd] -> Mux10/3
  [Simplex_Kp] -> Selector16/1, Selector15/1, Selector10/1
  Sum12/1 -> sigma/1
  sigma/1 -> Sum13/2
  Selector15/1 -> Sum12/2
  [mid_idx] -> Selector15/2
  [min_idx] -> Selector10/2
  [max_idx] -> Selector16/2
  sigma1/1 -> Sum15/2
  Sum14/1 -> sigma1/1
  Selector10/1 -> Sum12/1, Sum13/1, Sum15/1, Sum14/1
  Selector16/1 -> Sum14/2
  Sum13/1 -> [shr_Kp_mid]
  Sum15/1 -> [shr_Kp_max]
  Sum19/1 -> [shr_Kd_max]
  Sum17/1 -> [shr_Kd_mid]
  Selector19/1 -> Sum18/2
  Selector17/1 -> Sum18/1, Sum19/1, Sum17/1, Sum16/1
  Sum18/1 -> sigma3/1
  sigma3/1 -> Sum19/2
  [max_idx] -> Selector19/2
  [min_idx] -> Selector17/2
  [mid_idx] -> Selector18/2
  Selector18/1 -> Sum16/2
  sigma2/1 -> Sum17/2
  Sum16/1 -> sigma2/1
  [Simplex_Kd] -> Selector17/1, Selector18/1, Selector19/1
  [shr_Kp_mid] -> Mux8/2
  [shr_Kp_max] -> Mux8/3
  [shr_Kd_mid] -> Mux7/2
  [shr_Kd_max] -> Mux7/3
  [simplex_case] -> SimplexCase/1
